simulink model "HLCPlannerAndControllerTestBench"  (R2024b)
settings: Solver=VariableStepAuto  StartTime=0.0  StopTime=scenario.StopTime  FixedStep=Ts  RelTol=1e-3
PostLoadFcn:
  | helperSLHLCPlannerAndControllerSetup;
values from neighbouring files (symbols this model uses):
  mapInfo = struct('NumLanes', numLanes,'LaneWidth', zeros(maxNumLanes,1),                  'LaneCenters', zeros(maxNumLanes,1),'NumGlobalPlanPoints',                  size(globalPlanPoints,1), 'GlobalPlanPoints',                  zeros(maxGlobalPlanPoints,2))    [helperInitializeLaneChangeParameters.m]
  replanRate = 1    [helperInitializeLaneChangeParameters.m]
  timeHorizon = 1:3    [helperInitializeLaneChangeParameters.m]
  timeResolution = 0.1    [helperInitializeLaneChangeParameters.m]
undefined symbols (not defined in the file or in its folder): actorProfiles, egoFrontExt, egoTTC, enableCCBehavior, enableLCBehavior, enableLCFBehavior, frontSafetyGap, latDevCost, maxAccel, maxCurvature, maxPlanningHorizon, maxYawRate, minVelocity, nextTTC, preferredLane, rearSafetyGap, setSpeed, speedCost, targetFrontExt, timeCost, Ts
libraries: drivingscenarioandsensors x2
CloseFcn:
  | helperSLHLCPlannerAndControllerCleanUp;
settings Model: Creator=The MathWorks, Inc.  LastModifiedBy=The MathWorks, Inc.
settings SolverCC: ZeroCrossAlgorithm=Adaptive  AlgebraicLoopSolver=TrustRegion  MaxZcPerStep=1
settings DataIOCC: SaveOutput=off  ReturnWorkspaceOutputs=off
settings OptimizationCC: ReuseModelBlockBuffer=off
settings DebuggingCC: MaskedZcDiagnostic=none  IgnoredZcDiagnostic=none  UnconnectedInputMsg=warning  UnconnectedOutputMsg=warning  UnconnectedLineMsg=warning  SubsystemReferenceDiagnosticForUnitTest=warning
settings ModelReferenceCC: EnableRefExpFcnMdlSchedulingChecks=on
settings RTWCC: GPUComputeCapability=3.5  DLArmComputeVersion=19.05

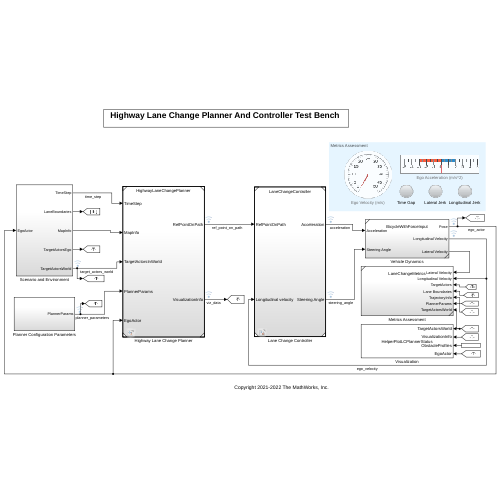
[thumbnail: Simulink's stored preview of the top-level diagram]
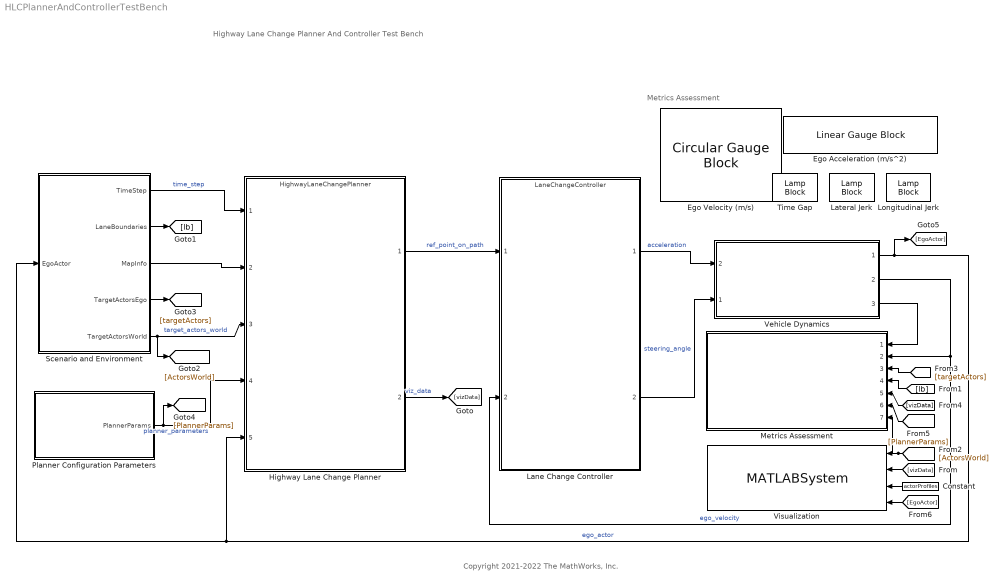
== system HLCPlannerAndControllerTestBench ==
  note: Copyright 2021-2022 The MathWorks, Inc.
  note: Metrics Assessment
  note: Highway Lane Change Planner And Controller Test Bench
  Constant : Constant  Value=actorProfiles  OutDataTypeStr=Bus: BusActorProfiles
  Ego Acceleration (m/s^2) : LinearGaugeBlock  LabelPosition=Hide  ScaleMin=-5  ScaleMax=5
  Ego Velocity (m/s) : CircularGaugeBlock  LabelPosition=Hide  ScaleMax=50  TickInterval=5
  Highway Lane Change Planner : ModelReference  ModelNameDialog=HighwayLaneChangePlanner.slx  SimulationMode=Normal  ModelReferenceVersion=10.0
  Lane Change Controller : ModelReference  ModelNameDialog=LaneChangeController.slx  SimulationMode=Normal  ModelReferenceVersion=9.0
  Lateral Jerk : LampBlock  LabelPosition=Hide
  Longitudinal Jerk : LampBlock  LabelPosition=Hide
  Metrics Assessment : Subsystem  ReferencedSubsystem=LaneChangeMetrics
  Planner Configuration Parameters : Subsystem
  Scenario and Environment : Subsystem
  Time Gap : LampBlock  LabelPosition=Hide
  Vehicle Dynamics : Subsystem  ReferencedSubsystem=BicycleWithForceInput
      settings: PortSchema="{\"entries\":[{\"content\":{\"sides\":[{\"content\":{\"connectorIds\":[\"In2\",\"In1\"]},\"type\":\"ConnectorPlacement.EquallySpacedRectSide\",\"uuid\":\"f63f66bc-f59a-4e63-885b-0681004bade6\"},{\"content\":{\"connectorIds\":[\"Out1\",\"Out2\",\"Out3\"],\"side\":\"RIGHT\"},\"type\":\"ConnectorPlacement.EquallySpacedRectSide\",\"uuid\":\"8ac8ea57-0210-4a13-ad95-4f0a9335ab33\"},{\"content\":{\"side\":\"TOP\"},\"type\":\"ConnectorPlacement.EquallySpacedRectSide\",\"uuid\":\"6d0b300d-41b2-47ad-8d2f-35db0d33cdc5\"}]},\"type\":\"ConnectorPlacement.EquallySpacedConnector\",\"uuid\":\"3215dd89-c688-4582-a904-15ea546ef61a\"}],\"packageUris\":[\"http://schema.mathworks.com/mf0/Connector/R2020b\"],\"version\":\"1.0\"}"
  Visualization : MATLABSystem  System=HelperPlotLCPlannerStatus  EnableTopView=on  EnableTrajTopView=on  EnableChaseView=on  EnableTrajChase=on  EnableCaplistChaseView=on
      mask Type: HelperPlotLCPlannerStatus
      mask Display:
      | disp('HelperPlotLCPlannerStatus');
      | port_label('input',1,'TargetActorsWorld');
      | port_label('input',2,'VisualizationInfo');
      | port_label('input',3,'ObstacleProfiles');
      | port_label('input',4,'EgoActor');
  wires:
  Planner Configuration Parameters/1(PlannerParams) -> [PlannerParams], Highway Lane Change Planner/4  "planner_parameters"
  Highway Lane Change Planner/2 -> [vizData]  "viz_data"
  [vizData] -> Visualization/2
  Scenario and Environment/2(LaneBoundaries) -> [lb]
  [lb] -> Metrics Assessment/4
  Highway Lane Change Planner/1 -> Lane Change Controller/1  "ref_point_on_path"
  [ActorsWorld] -> Metrics Assessment/7, Visualization/1
  Scenario and Environment/3(MapInfo) -> Highway Lane Change Planner/2
  Scenario and Environment/5(TargetActorsWorld) -> Highway Lane Change Planner/3, [ActorsWorld]  "target_actors_world"
  Scenario and Environment/4(TargetActorsEgo) -> [targetActors]
  Constant/1 -> Visualization/3
  [targetActors] -> Metrics Assessment/3
  Scenario and Environment/1(TimeStep) -> Highway Lane Change Planner/1  "time_step"
  Vehicle Dynamics/1 -> [EgoActor], Scenario and Environment/1(EgoActor), Highway Lane Change Planner/5  "ego_actor"
  Vehicle Dynamics/2 -> Lane Change Controller/2, Metrics Assessment/2  "ego_velocity"
  Vehicle Dynamics/3 -> Metrics Assessment/1
  Lane Change Controller/2 -> Vehicle Dynamics/1  "steering_angle"
  Lane Change Controller/1 -> Vehicle Dynamics/2  "acceleration"
  [vizData] -> Metrics Assessment/5
  [PlannerParams] -> Metrics Assessment/6
  [EgoActor] -> Visualization/4

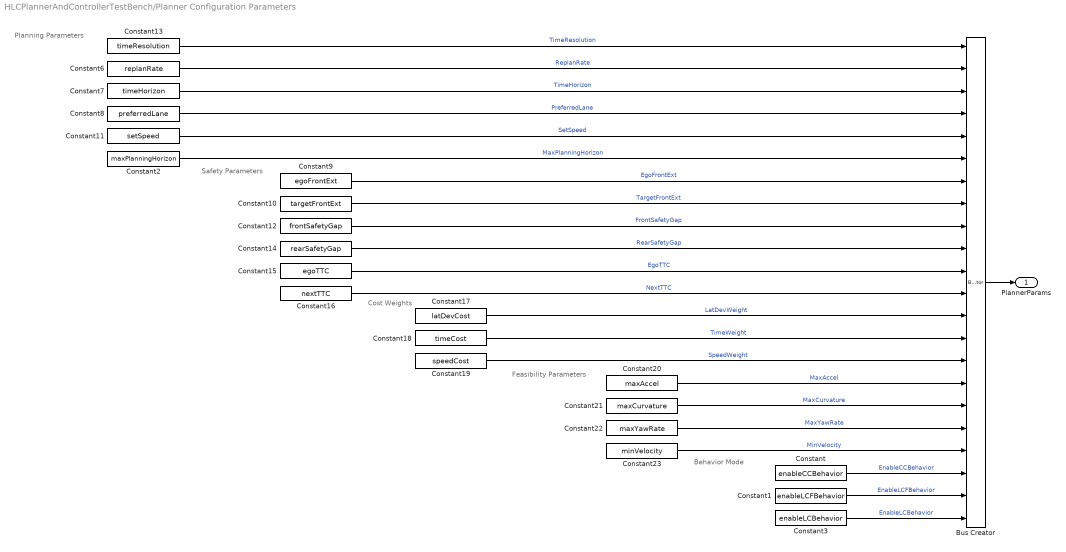
== system HLCPlannerAndControllerTestBench/Planner Configuration Parameters ==
  note: Planning Parameters
  note: Safety Parameters
  note: Cost Weights
  note: Feasibility Parameters
  note: Behavior Mode
  Bus Creator : BusCreator  Inputs=22  OutDataTypeStr=Bus: BusPlannerParams  NonVirtualBus=on
  Constant : Constant  Value=enableCCBehavior
  Constant1 : Constant  Value=enableLCFBehavior
  Constant10 : Constant  Value=targetFrontExt
  Constant11 : Constant  Value=setSpeed
  Constant12 : Constant  Value=frontSafetyGap
  Constant13 : Constant  Value=timeResolution
  Constant14 : Constant  Value=rearSafetyGap
  Constant15 : Constant  Value=egoTTC
  Constant16 : Constant  Value=nextTTC
  Constant17 : Constant  Value=latDevCost
  Constant18 : Constant  Value=timeCost
  Constant19 : Constant  Value=speedCost
  Constant2 : Constant  Value=maxPlanningHorizon
  Constant20 : Constant  Value=maxAccel
  Constant21 : Constant  Value=maxCurvature
  Constant22 : Constant  Value=maxYawRate
  Constant23 : Constant  Value=minVelocity
  Constant3 : Constant  Value=enableLCBehavior
  Constant6 : Constant  Value=replanRate
  Constant7 : Constant  Value=timeHorizon
  Constant8 : Constant  Value=preferredLane
  Constant9 : Constant  Value=egoFrontExt
  PlannerParams : Outport  OutDataTypeStr=Bus: BusPlannerParams
  wires:
  Constant19/1 -> Bus Creator/15  "SpeedWeight"
  Constant15/1 -> Bus Creator/11  "EgoTTC"
  Constant12/1 -> Bus Creator/9  "FrontSafetyGap"
  Constant6/1 -> Bus Creator/2  "ReplanRate"
  Constant14/1 -> Bus Creator/10  "RearSafetyGap"
  Constant20/1 -> Bus Creator/16  "MaxAccel"
  Constant18/1 -> Bus Creator/14  "TimeWeight"
  Constant11/1 -> Bus Creator/5  "SetSpeed"
  Constant13/1 -> Bus Creator/1  "TimeResolution"
  Constant23/1 -> Bus Creator/19  "MinVelocity"
  Constant9/1 -> Bus Creator/7  "EgoFrontExt"
  Constant16/1 -> Bus Creator/12  "NextTTC"
  Constant10/1 -> Bus Creator/8  "TargetFrontExt"
  Constant7/1 -> Bus Creator/3  "TimeHorizon"
  Constant21/1 -> Bus Creator/17  "MaxCurvature"
  Constant8/1 -> Bus Creator/4  "PreferredLane"
  Constant17/1 -> Bus Creator/13  "LatDevWeight"
  Bus Creator/1 -> PlannerParams/1
  Constant22/1 -> Bus Creator/18  "MaxYawRate"
  Constant/1 -> Bus Creator/20  "EnableCCBehavior"
  Constant1/1 -> Bus Creator/21  "EnableLCFBehavior"
  Constant3/1 -> Bus Creator/22  "EnableLCBehavior"
  Constant2/1 -> Bus Creator/6  "MaxPlanningHorizon"

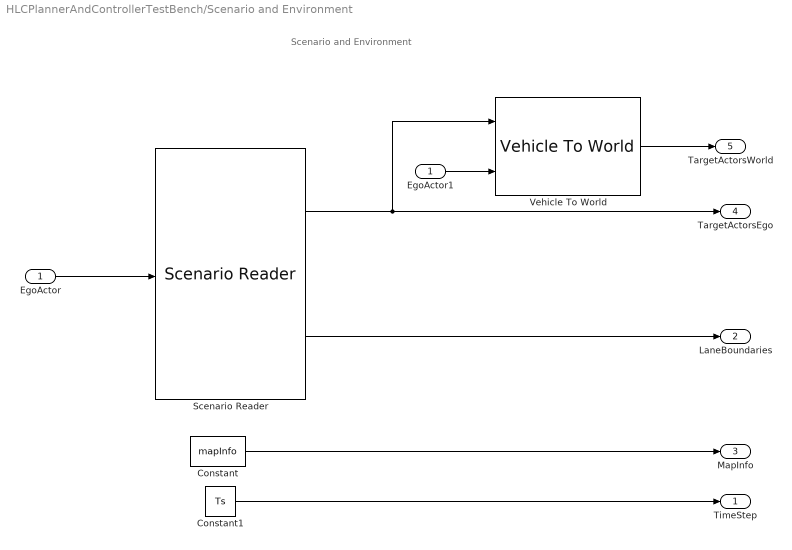
== system HLCPlannerAndControllerTestBench/Scenario and Environment ==
  note: Scenario and Environment
  EgoActor : Inport
  Constant : Constant  Value=mapInfo  OutDataTypeStr=Bus: BusMapInfo
  Constant1 : Constant  Value=Ts
  EgoActor1 : InportShadow
  Scenario Reader : drivingscenarioandsensors/Scenario Reader  ScenarioSource=From workspace  ScenarioFileName=CurevedRoadNetwork.mat  ScenarioVariableName=scenario  OutputCoordinateSystem=Vehicle coordinates  EgoVehicleSource=Input port  EgoVehicleActorID=egoInitialPose.ActorID  OrientVehiclesOnRoad=off  OutputEgoVehiclePose=off  OutputEgoVehicleState=off  SampleTime=0.1  LaneBoundaryOutput=Ego vehicle lane boundaries  LaneBoundaryDistance=0:0.5:60  LaneBoundaryLocation=Center of lane markings  BusNameSource=Property  BusName=BusActorsTruth  BusNumActorsSource=Scenario  BusNumActors=100  BusName2Source=Auto  BusName2=BusLaneBoundaries  BusNumLaneBoundariesSource=Scenario  BusNumLaneBoundaries=10  BusName3Source=Auto  BusName3=BusEgoActor  BusName4Source=Auto  BusName4=BusEgoState  ShowCoordinateLabels=on  SimulateUsing=Interpreted execution
  Vehicle To World : drivingscenarioandsensors/Vehicle To World  BusNameSource=Property  BusName=BusActorsEgo  SimulateUsing=Interpreted execution
  TimeStep : Outport
  LaneBoundaries : Outport  Port=2
  MapInfo : Outport  Port=3  OutDataTypeStr=Bus: BusMapInfo
  TargetActorsEgo : Outport  Port=4  VectorParamsAs1DForOutWhenUnconnected=off
  TargetActorsWorld : Outport  Port=5
  wires:
  EgoActor/1 -> Scenario Reader/1
  Scenario Reader/1 -> Vehicle To World/1, TargetActorsEgo/1
  Scenario Reader/2 -> LaneBoundaries/1
  Constant/1 -> MapInfo/1
  EgoActor1/1 -> Vehicle To World/2
  Vehicle To World/1 -> TargetActorsWorld/1
  Constant1/1 -> TimeStep/1
